simulink model "Modified_Step"  (R2023a)
settings: Solver=VariableStepAuto  StartTime=0.0  StopTime=10.0  RelTol=1e-3
values from neighbouring files (symbols this model uses):
  B = 30.2*0.137*60/(1000*7580*2*pi)    (= 5.21230338957e-06)    [Mechatronics.m]
  J = 142/(1000*100*100)    (= 1.42e-05)    [Mechatronics.m]
  Kp = 1    [Mechatronics.m]
  Kt = 30.2/1000    (= 0.0302)    [Mechatronics.m]
  Kw = 60/(317*2*pi)    (= 0.0301239639922)    [Mechatronics.m]
  L = 0.0823/1000    (= 8.23e-05)    [Mechatronics.m]
  R = 0.299    [Mechatronics.m]
undefined symbols (not defined in the file or in its folder): Ki
settings Model: Creator=karteek  LastModifiedBy=karteek

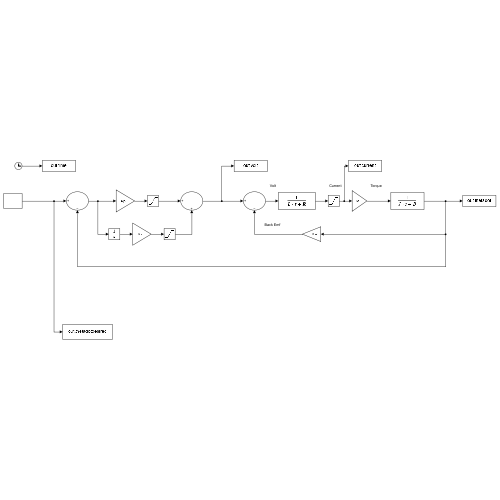
[thumbnail: Simulink's stored preview of the top-level diagram]
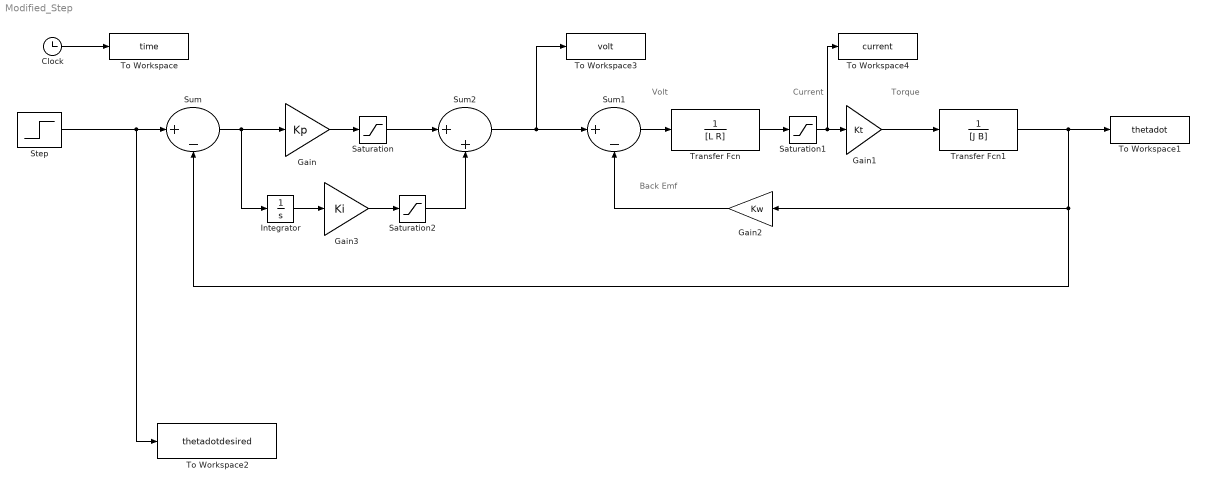
== system Modified_Step ==
  note: Volt
  note: Torque
  note: Current
  note: Back Emf
  Clock : Clock
  Gain : Gain  Gain=Kp
  Gain1 : Gain  Gain=Kt
  Gain2 : Gain  Gain=Kw
  Gain3 : Gain  Gain=Ki
  Integrator : Integrator
  Saturation : Saturate  UpperLimit=24  LowerLimit=-24
  Saturation1 : Saturate  UpperLimit=80  LowerLimit=-80
  Saturation2 : Saturate  UpperLimit=24  LowerLimit=-24
  Step : Step  After=4000*2*pi/60  SampleTime=0
  Sum : Sum  Inputs=|+-
  Sum1 : Sum  Inputs=|+-
  Sum2 : Sum  Inputs=|++
  To Workspace : ToWorkspace  VariableName=time  SampleTime=-1
  To Workspace1 : ToWorkspace  VariableName=thetadot  SampleTime=-1
  To Workspace2 : ToWorkspace  VariableName=thetadotdesired  SampleTime=-1
  To Workspace3 : ToWorkspace  VariableName=volt  SampleTime=-1
  To Workspace4 : ToWorkspace  VariableName=current  SampleTime=-1
  Transfer Fcn : TransferFcn  Denominator=[L R]
  Transfer Fcn1 : TransferFcn  Denominator=[J B]
  wires:
  Sum1/1 -> Transfer Fcn/1
  Clock/1 -> To Workspace/1
  Sum/1 -> Integrator/1, Gain/1
  Gain/1 -> Saturation/1
  Transfer Fcn1/1 -> Gain2/1, Sum/2, To Workspace1/1
  Gain2/1 -> Sum1/2
  Step/1 -> Sum/1, To Workspace2/1
  Gain1/1 -> Transfer Fcn1/1
  Transfer Fcn/1 -> Saturation1/1
  Saturation1/1 -> To Workspace4/1, Gain1/1
  Saturation/1 -> Sum2/1
  Sum2/1 -> To Workspace3/1, Sum1/1
  Integrator/1 -> Gain3/1
  Gain3/1 -> Saturation2/1
  Saturation2/1 -> Sum2/2
